simulink model "Direct_D_z"  (R2018b)
settings: Solver=VariableStepAuto  StartTime=0.0  StopTime=10  RelTol=1e-3
settings Model: Creator=LEGION  LastModifiedBy=LEGION

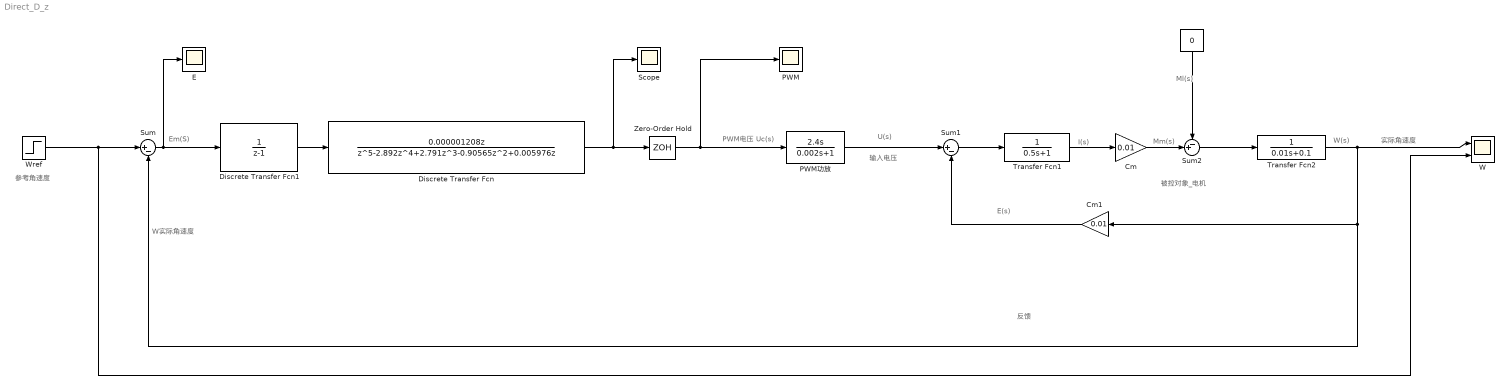
== system Direct_D_z ==
  note: 反馈
  note: 被控对象_电机
  note: W实际角速度
  note: U(s)
  note: Ml(s)
  note: 参考角速度
  note: I(s)
  note: PWM电压 Uc(s)
  note: W(s)
  note: 输入电压
  note: E(s)
  note: Em(S)
  note: 实际角速度
  note: Mm(s)
  " " : Constant  Value=0
  Cm : Gain  Gain=0.01
  Cm1 : Gain  Gain=0.01
  Discrete Transfer Fcn : DiscreteTransferFcn  Numerator=[0.000001208 0]  Denominator=[1 -2.892 2.791 -0.90565 0.005976 0]  SampleTime=0.05
  Discrete Transfer Fcn1 : DiscreteTransferFcn  Denominator=[1 -1]  SampleTime=0.05
  E : Scope
  PWM : Scope
  PWM功放 : TransferFcn  Numerator=[2.4 0]  Denominator=[0.002 1]
  Scope : Scope
  Sum : Sum  Inputs=|+-
  Sum1 : Sum  Inputs=|+-
  Sum2 : Sum  Inputs=-+|
  Transfer Fcn1 : TransferFcn  Denominator=[0.5 1]
  Transfer Fcn2 : TransferFcn  Denominator=[0.01 0.1]
  W : Scope  NumInputPorts=2
  Wref : Step  Time=0  SampleTime=0
  Zero-Order Hold : ZeroOrderHold  SampleTime=0.05
  wires:
  " "/1 -> Sum2/1
  Cm/1 -> Sum2/2
  Sum1/1 -> Transfer Fcn1/1
  Transfer Fcn2/1 -> Sum/2, Cm1/1, W/1
  PWM功放/1 -> Sum1/1
  Transfer Fcn1/1 -> Cm/1
  Sum/1 -> Discrete Transfer Fcn1/1, E/1
  Zero-Order Hold/1 -> PWM/1, PWM功放/1
  Wref/1 -> Sum/1, W/2
  Sum2/1 -> Transfer Fcn2/1
  Cm1/1 -> Sum1/2
  Discrete Transfer Fcn/1 -> Scope/1, Zero-Order Hold/1
  Discrete Transfer Fcn1/1 -> Discrete Transfer Fcn/1
